simulink model "gm_simpleController_vnl"  (R2020b)
settings: Solver=FixedStepDiscrete  StartTime=0.0  StopTime=10.0  RelTol=1e-3
libraries: hdlmdlgenlib x8, simulink x2
settings Model: Creator=amira  LastModifiedBy=amira
settings OptimizationCC: BlockReduction=off  ConditionallyExecuteInputs=off
settings DebuggingCC: InheritedTsInSrcMsg=none

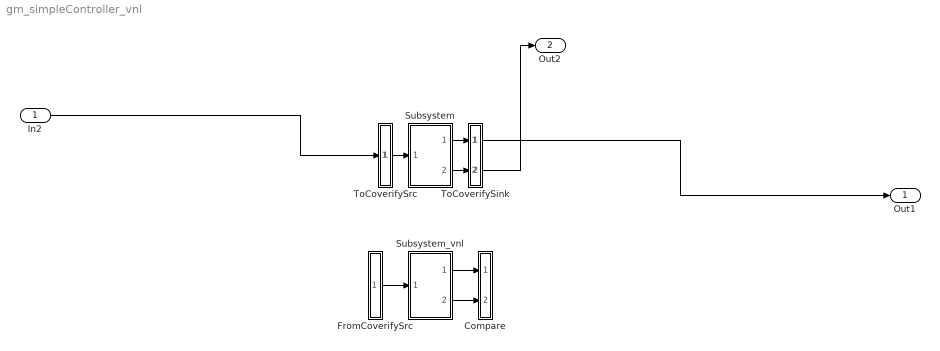
== system gm_simpleController_vnl ==
  In2 : Inport
  Compare : Subsystem
      mask Display: disp('')
  FromCoverifySrc : Subsystem
      mask Display: disp('')
  Subsystem : Subsystem
  Subsystem_vnl : Subsystem
  ToCoverifySink : Subsystem
      mask Display: disp('')
  ToCoverifySrc : Subsystem
      mask Display: disp('')
  Out1 : Outport  SignalName=C  VectorParamsAs1DForOutWhenUnconnected=off
  Out2 : Outport  Port=2  SignalName=U  VectorParamsAs1DForOutWhenUnconnected=off
  wires:
  ToCoverifySrc/1(out1) -> Subsystem/1(In2)
  Subsystem/1(Out1) -> ToCoverifySink/1(in1)
  Subsystem/2(Out2) -> ToCoverifySink/2(in2)
  In2/1 -> ToCoverifySrc/1(in1)
  ToCoverifySink/1(out1) -> Out1/1
  ToCoverifySink/2(out2) -> Out2/1
  FromCoverifySrc/1(out1) -> Subsystem_vnl/1(In2)
  Subsystem_vnl/1(Out1) -> Compare/1(in1)
  Subsystem_vnl/2(Out2) -> Compare/2(in2)

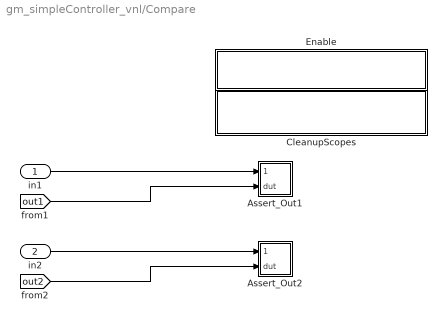
== system gm_simpleController_vnl/Compare ==
  in1 : Inport
  in2 : Inport  Port=2
  Assert_Out1 : Subsystem  mask{ToleranceValue=1e-07}
  Assert_Out2 : Subsystem  mask{ToleranceValue=1e-07}
  CleanupScopes : Subsystem
      settings: OpenFcn=|
      | blkName = gcb; %self block
      | idx = regexp(blkName, '/CleanupScopes$', 'once');
      | blkParent = blkName(1:idx-1);
      | blks=find_system(blkParent, 'LookUnderMasks', 'all','blocktype', 'Scope');
      | for itr = 1:length(blks)
      | 	 hScopeCfg = get_param(blks{itr},'ScopeConfiguration');
      | 	 hScopeCfg.Visible = ~ hScopeCfg.Visible;
      | end
      | drawnow;
      mask Display: fprintf(message('hdlcoder:cosim:vnl_dblclick').getString());
  Enable : Subsystem
      settings: OpenFcn=|
      | blkName = gcb;
      | idx = regexp(blkName, '/Enable$', 'once');
      | blkParent = blkName(1:idx-1);
      | blks=find_system(blkParent, 'LookUnderMasks', 'all','blocktype', 'Assertion');
      | e = get_param(blks{1}, 'Enabled');
      | if strcmp(e, 'on'), f= 'off';, else, f = 'on';, end
      | for ii=1:length(blks), set_param(blks{ii}, 'Enabled', f);, end
      | set_param(gcb, 'MaskDisplay',['fprintf(message(''hdlcoder:cosim:vnl_dblclick_assertions'',','''',upper(e),'''',').getString())']);
      mask Display: fprintf(message('hdlcoder:cosim:vnl_dblclick_assertions','OFF').getString());
  wires:
  in1/1 -> Assert_Out1/1(cosim)
  [out1] -> Assert_Out1/2(dut)
  in2/1 -> Assert_Out2/1(cosim)
  [out2] -> Assert_Out2/2(dut)

== system gm_simpleController_vnl/FromCoverifySrc ==
  out1 : Outport
  wires:
  [in1] -> out1/1

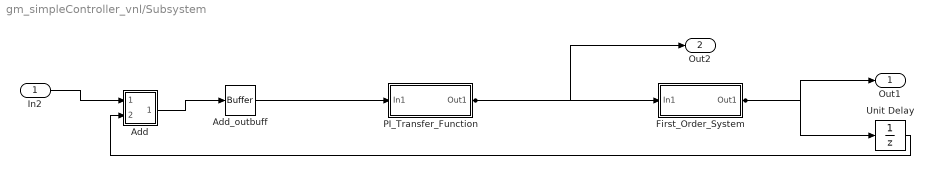
== system gm_simpleController_vnl/Subsystem ==
  In2 : Inport  OutDataTypeStr=single  PortDimensions=1  SampleTime=0.2
  Add : Subsystem
      mask Display: disp('NFP\nadd');
  Add_outbuff : hdlmdlgenlib/Buffer
      settings: SourceProductBaseCode=SL
  First_Order_System : Subsystem
  PI_Transfer_Function : Subsystem
  Unit Delay : UnitDelay  InitialCondition=single(0)  SampleTime=0.2
  Out1 : Outport  OutDataTypeStr=single  VectorParamsAs1DForOutWhenUnconnected=off
  Out2 : Outport  Port=2  OutDataTypeStr=single  VectorParamsAs1DForOutWhenUnconnected=off
  wires:
  Add/1(Out1) -> Add_outbuff/1
  Unit Delay/1 -> Add/2(In2)
  PI_Transfer_Function/1(Out1) -> First_Order_System/1(In1), Out2/1
  First_Order_System/1(Out1) -> Out1/1, Unit Delay/1
  Add_outbuff/1 -> PI_Transfer_Function/1(In1)
  In2/1 -> Add/1(In1)

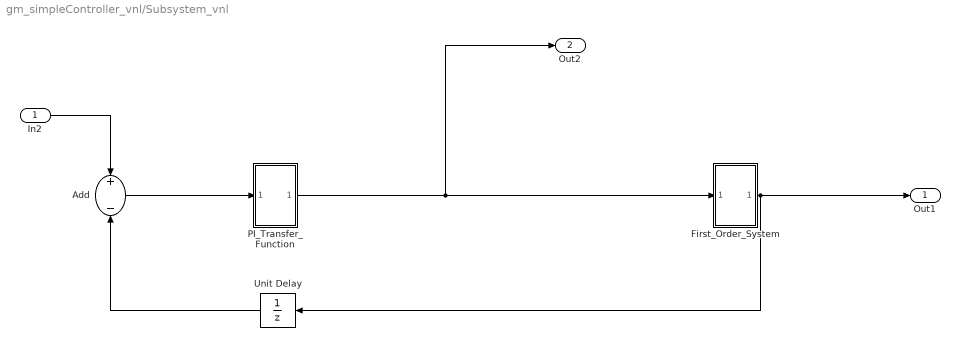
== system gm_simpleController_vnl/Subsystem_vnl ==
  In2 : Inport  OutDataTypeStr=single
  Add : Sum  Inputs=+-  AccumDataTypeStr=single
  First_Order_System : Subsystem
  PI_Transfer_Function : Subsystem
  Unit Delay : UnitDelay  SampleTime=-1  HasFrameUpgradeWarning=on
  Out1 : Outport  OutDataTypeStr=single  VectorParamsAs1DForOutWhenUnconnected=off
  Out2 : Outport  Port=2  OutDataTypeStr=single  VectorParamsAs1DForOutWhenUnconnected=off
  wires:
  Unit Delay/1 -> Add/2
  Add/1 -> PI_Transfer_Function/1(In1)
  PI_Transfer_Function/1(Out1) -> First_Order_System/1(In1), Out2/1
  First_Order_System/1(Out1) -> Out1/1, Unit Delay/1
  In2/1 -> Add/1

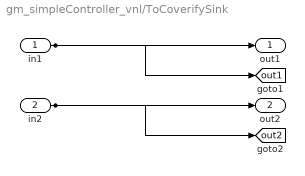
== system gm_simpleController_vnl/ToCoverifySink ==
  in1 : Inport
  in2 : Inport  Port=2
  out1 : Outport
  out2 : Outport  Port=2
  tag scope: out1=global, out2=global
  wires:
  in1/1 -> out1/1, [out1]
  in2/1 -> out2/1, [out2]

== system gm_simpleController_vnl/ToCoverifySrc ==
  in1 : Inport
  out1 : Outport
  tag scope: in1=global
  wires:
  in1/1 -> out1/1, [in1]

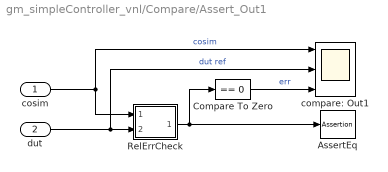
== system gm_simpleController_vnl/Compare/Assert_Out1 ==
  cosim : Inport
  dut : Inport  Port=2
  AssertEq : Assertion  StopWhenAssertionFail=off
  Compare To Zero : simulink/Logic and Bit Operations/Compare To Zero  relop===  OutDataTypeStr=boolean
  RelErrCheck : Subsystem
  compare: Out1 : Scope  NumInputPorts=3
  wires:
  dut/1 -> compare: Out1/2, RelErrCheck/2(In2)  "dut ref"
  cosim/1 -> compare: Out1/1, RelErrCheck/1(In1)  "cosim"
  RelErrCheck/1(Out1) -> AssertEq/1, Compare To Zero/1
  Compare To Zero/1 -> compare: Out1/3  "err"

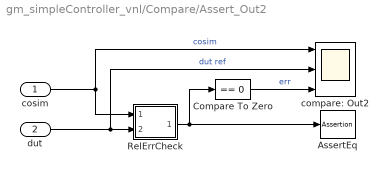
== system gm_simpleController_vnl/Compare/Assert_Out2 ==
  cosim : Inport
  dut : Inport  Port=2
  AssertEq : Assertion  StopWhenAssertionFail=off
  Compare To Zero : simulink/Logic and Bit Operations/Compare To Zero  relop===  OutDataTypeStr=boolean
  RelErrCheck : Subsystem
  compare: Out2 : Scope  NumInputPorts=3
  wires:
  dut/1 -> compare: Out2/2, RelErrCheck/2(In2)  "dut ref"
  cosim/1 -> compare: Out2/1, RelErrCheck/1(In1)  "cosim"
  RelErrCheck/1(Out1) -> AssertEq/1, Compare To Zero/1
  Compare To Zero/1 -> compare: Out2/3  "err"

== system gm_simpleController_vnl/Compare/CleanupScopes ==

== system gm_simpleController_vnl/Compare/Enable ==

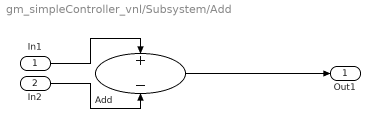
== system gm_simpleController_vnl/Subsystem/Add ==
  In1 : Inport
  In2 : Inport  Port=2
  Add : Sum  Inputs=+-  OutDataTypeStr=single  SampleTime=0.2
  Out1 : Outport
  wires:
  Add/1 -> Out1/1
  In2/1 -> Add/2
  In1/1 -> Add/1

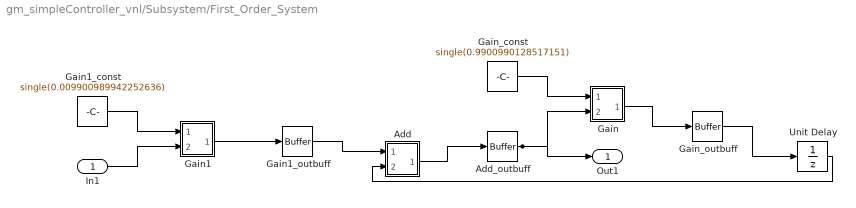
== system gm_simpleController_vnl/Subsystem/First_Order_System ==
  In1 : Inport  OutDataTypeStr=single  PortDimensions=1  SampleTime=0.2
  Add : Subsystem
      mask Display: disp('NFP\nadd');
  Add_outbuff : hdlmdlgenlib/Buffer
      settings: SourceProductBaseCode=SL
  Gain : Subsystem
      mask Display: disp('NFP\nmul');
  Gain1 : Subsystem
      mask Display: disp('NFP\nmul');
  Gain1_const : Constant  Value=single(0.009900989942252636)  OutDataTypeStr=single  SampleTime=0.2
  Gain1_outbuff : hdlmdlgenlib/Buffer
      settings: SourceProductBaseCode=SL
  Gain_const : Constant  Value=single(0.9900990128517151)  OutDataTypeStr=single  SampleTime=0.2
  Gain_outbuff : hdlmdlgenlib/Buffer
      settings: SourceProductBaseCode=SL
  Unit Delay : UnitDelay  InitialCondition=single(0)  SampleTime=0.2
  Out1 : Outport  VectorParamsAs1DForOutWhenUnconnected=off
  wires:
  Gain1/1(Out1) -> Gain1_outbuff/1
  Gain/1(Out1) -> Gain_outbuff/1
  Add/1(Out1) -> Add_outbuff/1
  Gain1_const/1 -> Gain1/1(In1)
  Gain_const/1 -> Gain/1(In1)
  Unit Delay/1 -> Add/2(In2)
  Gain1_outbuff/1 -> Add/1(In1)
  Gain_outbuff/1 -> Unit Delay/1
  Add_outbuff/1 -> Out1/1, Gain/2(In2)
  In1/1 -> Gain1/2(In2)

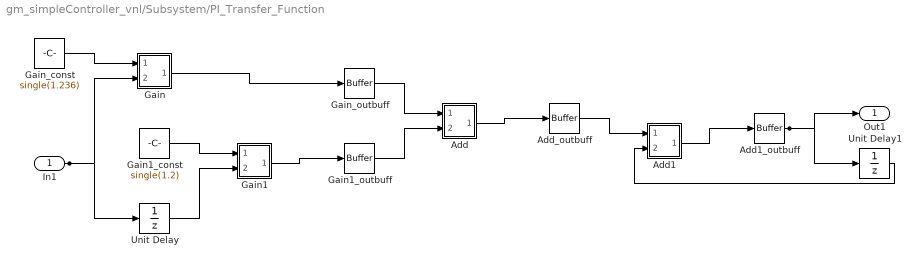
== system gm_simpleController_vnl/Subsystem/PI_Transfer_Function ==
  In1 : Inport  OutDataTypeStr=single  PortDimensions=1  SampleTime=0.2
  Add : Subsystem
      mask Display: disp('NFP\nadd');
  Add1 : Subsystem
      mask Display: disp('NFP\nadd');
  Add1_outbuff : hdlmdlgenlib/Buffer
      settings: SourceProductBaseCode=SL
  Add_outbuff : hdlmdlgenlib/Buffer
      settings: SourceProductBaseCode=SL
  Gain : Subsystem
      mask Display: disp('NFP\nmul');
  Gain1 : Subsystem
      mask Display: disp('NFP\nmul');
  Gain1_const : Constant  Value=single(1.2)  OutDataTypeStr=single  SampleTime=0.2
  Gain1_outbuff : hdlmdlgenlib/Buffer
      settings: SourceProductBaseCode=SL
  Gain_const : Constant  Value=single(1.236)  OutDataTypeStr=single  SampleTime=0.2
  Gain_outbuff : hdlmdlgenlib/Buffer
      settings: SourceProductBaseCode=SL
  Unit Delay : UnitDelay  InitialCondition=single(0)  SampleTime=0.2
  Unit Delay1 : UnitDelay  InitialCondition=single(0)  SampleTime=0.2
  Out1 : Outport  VectorParamsAs1DForOutWhenUnconnected=off
  wires:
  Gain1/1(Out1) -> Gain1_outbuff/1
  Gain/1(Out1) -> Gain_outbuff/1
  Add1/1(Out1) -> Add1_outbuff/1
  Add/1(Out1) -> Add_outbuff/1
  Gain1_const/1 -> Gain1/1(In1)
  Gain_const/1 -> Gain/1(In1)
  Unit Delay1/1 -> Add1/2(In2)
  Unit Delay/1 -> Gain1/2(In2)
  Gain1_outbuff/1 -> Add/2(In2)
  Gain_outbuff/1 -> Add/1(In1)
  Add1_outbuff/1 -> Out1/1, Unit Delay1/1
  Add_outbuff/1 -> Add1/1(In1)
  In1/1 -> Unit Delay/1, Gain/2(In2)

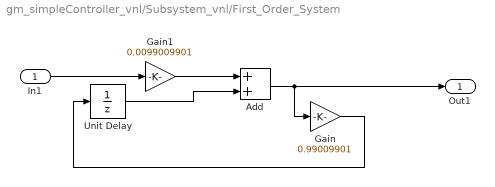
== system gm_simpleController_vnl/Subsystem_vnl/First_Order_System ==
  In1 : Inport
  Add : Sum  AccumDataTypeStr=single
  Gain : Gain  Gain=0.99009901  ParamDataTypeStr=single  OutDataTypeStr=single
  Gain1 : Gain  Gain=0.0099009901  ParamDataTypeStr=single  OutDataTypeStr=single
  Unit Delay : UnitDelay  SampleTime=-1  HasFrameUpgradeWarning=on
  Out1 : Outport  VectorParamsAs1DForOutWhenUnconnected=off
  wires:
  Add/1 -> Gain/1, Out1/1
  Unit Delay/1 -> Add/2
  In1/1 -> Gain1/1
  Gain1/1 -> Add/1
  Gain/1 -> Unit Delay/1

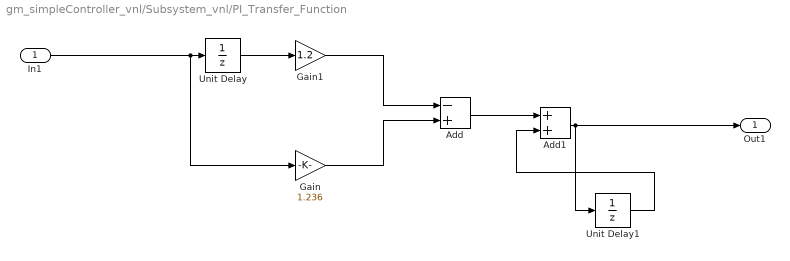
== system gm_simpleController_vnl/Subsystem_vnl/PI_Transfer_Function ==
  In1 : Inport
  Add : Sum  Inputs=-+  AccumDataTypeStr=single
  Add1 : Sum  AccumDataTypeStr=single
  Gain : Gain  Gain=1.236  ParamDataTypeStr=single  OutDataTypeStr=single
  Gain1 : Gain  Gain=1.2  ParamDataTypeStr=single  OutDataTypeStr=single
  Unit Delay : UnitDelay  SampleTime=-1  HasFrameUpgradeWarning=on
  Unit Delay1 : UnitDelay  SampleTime=-1  HasFrameUpgradeWarning=on
  Out1 : Outport  VectorParamsAs1DForOutWhenUnconnected=off
  wires:
  Add/1 -> Add1/1
  In1/1 -> Unit Delay/1, Gain/1
  Gain/1 -> Add/2
  Unit Delay1/1 -> Add1/2
  Gain1/1 -> Add/1
  Add1/1 -> Unit Delay1/1, Out1/1
  Unit Delay/1 -> Gain1/1

== system gm_simpleController_vnl/Compare/Assert_Out1/RelErrCheck ==
  In1 : Inport
  In2 : Inport  Port=2
  "RelativeErrorCheck " : MATLAB Function  TreatAsAtomicUnit=on
  Out1 : Outport  VectorParamsAs1DForOutWhenUnconnected=off
  wires:
  In2/1 -> "RelativeErrorCheck "/2(R)
  In1/1 -> "RelativeErrorCheck "/1(P)
  "RelativeErrorCheck "/1(y) -> Out1/1

== system gm_simpleController_vnl/Compare/Assert_Out2/RelErrCheck ==
  In1 : Inport
  In2 : Inport  Port=2
  "RelativeErrorCheck " : MATLAB Function  TreatAsAtomicUnit=on
  Out1 : Outport  VectorParamsAs1DForOutWhenUnconnected=off
  wires:
  In2/1 -> "RelativeErrorCheck "/2(R)
  In1/1 -> "RelativeErrorCheck "/1(P)
  "RelativeErrorCheck "/1(y) -> Out1/1

== system gm_simpleController_vnl/Subsystem/First_Order_System/Add ==
  In1 : Inport
  In2 : Inport  Port=2
  Add : Sum  OutDataTypeStr=single  SampleTime=0.2
  Out1 : Outport
  wires:
  Add/1 -> Out1/1
  In2/1 -> Add/2
  In1/1 -> Add/1

== system gm_simpleController_vnl/Subsystem/First_Order_System/Gain ==
  In1 : Inport
  In2 : Inport  Port=2
  Gain : Product  Inputs=**  OutDataTypeStr=single  SampleTime=0.2
  Out1 : Outport
  wires:
  Gain/1 -> Out1/1
  In2/1 -> Gain/2
  In1/1 -> Gain/1

== system gm_simpleController_vnl/Subsystem/First_Order_System/Gain1 ==
  In1 : Inport
  In2 : Inport  Port=2
  Gain1 : Product  Inputs=**  OutDataTypeStr=single  SampleTime=0.2
  Out1 : Outport
  wires:
  Gain1/1 -> Out1/1
  In2/1 -> Gain1/2
  In1/1 -> Gain1/1

== system gm_simpleController_vnl/Subsystem/PI_Transfer_Function/Add ==
  In1 : Inport
  In2 : Inport  Port=2
  Add : Sum  Inputs=+-  OutDataTypeStr=single  SampleTime=0.2
  Out1 : Outport
  wires:
  Add/1 -> Out1/1
  In2/1 -> Add/2
  In1/1 -> Add/1

== system gm_simpleController_vnl/Subsystem/PI_Transfer_Function/Add1 ==
  In1 : Inport
  In2 : Inport  Port=2
  Add1 : Sum  OutDataTypeStr=single  SampleTime=0.2
  Out1 : Outport
  wires:
  Add1/1 -> Out1/1
  In2/1 -> Add1/2
  In1/1 -> Add1/1

== system gm_simpleController_vnl/Subsystem/PI_Transfer_Function/Gain ==
  In1 : Inport
  In2 : Inport  Port=2
  Gain : Product  Inputs=**  OutDataTypeStr=single  SampleTime=0.2
  Out1 : Outport
  wires:
  Gain/1 -> Out1/1
  In2/1 -> Gain/2
  In1/1 -> Gain/1

== system gm_simpleController_vnl/Subsystem/PI_Transfer_Function/Gain1 ==
  In1 : Inport
  In2 : Inport  Port=2
  Gain1 : Product  Inputs=**  OutDataTypeStr=single  SampleTime=0.2
  Out1 : Outport
  wires:
  Gain1/1 -> Out1/1
  In2/1 -> Gain1/2
  In1/1 -> Gain1/1

== matlab function gm_simpleController_vnl/Compare/Assert_Out1/RelErrCheck/RelativeErrorCheck  ==
  data: P input; y output; R input; ToleranceValue parameter double
% Check if the relative error of R with respect to P is below
% ToleranceValue
% P, R are floating-point
function y = relErrCheck(P,R, ToleranceValue)
    tol = ToleranceValue;
    sz = numel(P);
    assert(sz == numel(R), 'Inputs P and R have different sizes.');
    y = false(1, sz);

    for ii=1:sz
        if (isnan(P(ii)) || isnan(R(ii)))
            if (isnan(P(ii)) && isnan(R(ii)))
                y(ii) = true;
            end
        elseif (isinf(P(ii)) || isinf(R(ii)))
            y(ii) = (P(ii) == R(ii));
        elseif (P(ii) == 0)
            y(ii) = (R(ii) == 0);
        else
            absdiff = abs(P(ii) - R(ii));
            relerr = absdiff/abs(P(ii));
            y(ii) = (relerr <= tol);
        end
    end
end

== matlab function gm_simpleController_vnl/Compare/Assert_Out2/RelErrCheck/RelativeErrorCheck  ==
  data: P input; y output; R input; ToleranceValue parameter double
% Check if the relative error of R with respect to P is below
% ToleranceValue
% P, R are floating-point
function y = relErrCheck(P,R, ToleranceValue)
    tol = ToleranceValue;
    sz = numel(P);
    assert(sz == numel(R), 'Inputs P and R have different sizes.');
    y = false(1, sz);

    for ii=1:sz
        if (isnan(P(ii)) || isnan(R(ii)))
            if (isnan(P(ii)) && isnan(R(ii)))
                y(ii) = true;
            end
        elseif (isinf(P(ii)) || isinf(R(ii)))
            y(ii) = (P(ii) == R(ii));
        elseif (P(ii) == 0)
            y(ii) = (R(ii) == 0);
        else
            absdiff = abs(P(ii) - R(ii));
            relerr = absdiff/abs(P(ii));
            y(ii) = (relerr <= tol);
        end
    end
end
